simulink model "fftTest"  (R2020b)
settings: Solver=FixedStepDiscrete  StartTime=0.0  StopTime=stopTime  RelTol=1e-3
PostLoadFcn:
  | addpath([fileparts(which(bdroot)) filesep '..' filesep])
InitFcn:
  | simulinkInitFFT
StopFcn:
  | simulinkVerifyFFT
undefined symbols (not defined in the file or in its folder): params
libraries: dspsrcs4 x1
settings Model: DataTypeOverride=Off  SimulationMode=accelerator  Creator=trevor  LastModifiedBy=trevor
settings DataIOCC: SaveFormat=Array  SaveOutput=off  DSMLogging=off  SaveTime=off  ReturnWorkspaceOutputs=off
settings OptimizationCC: BlockReduction=off  ConditionallyExecuteInputs=off  DefaultParameterBehavior=Inlined
settings DebuggingCC: AlgebraicLoopMsg=error  SingleTaskRateTransMsg=error  SFMachineParentedDataDiag=error
settings HardwareCC: ProdBitPerPointer=32  ProdBitPerSizeT=32  ProdBitPerPtrDiffT=32  ProdLargestAtomicFloat=None  ProdIntDivRoundTo=Undefined  ProdEndianess=Unspecified  ProdWordSize=32  ProdHWDeviceType=ASIC/FPGA->ASIC/FPGA  TargetBitPerLong=64  TargetBitPerPointer=64  TargetBitPerSizeT=64  TargetBitPerPtrDiffT=64  TargetLongLongMode=on  TargetIntDivRoundTo=Zero  TargetEndianess=LittleEndian  TargetWordSize=64  TargetHWDeviceType=Custom Processor->MATLAB Host Computer  ProdEqTarget=off

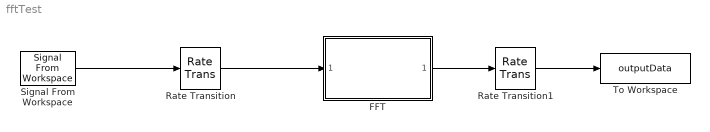
== system fftTest ==
  FFT : Subsystem  ReferencedSubsystem=FFT
  Rate Transition : RateTransition  Deterministic=off  OutPortSampleTime=params.systemClockPeriod
  Rate Transition1 : RateTransition  OutPortSampleTime=params.samplingPeriod
  Signal From Workspace : dspsrcs4/Signal From Workspace  X=testData  Ts=params.samplingPeriod  nsamps=1  OutputAfterFinalValue=Setting to zero  ignoreOrWarnInputAndFrameLengths=off  OutputFrames=off
  To Workspace : ToWorkspace  VariableName=outputData  SampleTime=-1
      settings: Save2DSignal=2-D array (concatenate along first dimension)
  wires:
  FFT/1 -> Rate Transition1/1
  Signal From Workspace/1 -> Rate Transition/1
  Rate Transition/1 -> FFT/1
  Rate Transition1/1 -> To Workspace/1
